simulink model "linearModel"  (R2019a)
settings: Solver=ode45  StartTime=0.0  StopTime=SimulationTime  MaxStep=maxstep  RelTol=rtol
undefined symbols (not defined in the file or in its folder): A, B, beta_operating, C, D, deviation, ePhi, operatingPoint
libraries: simulink x1
settings Model: Creator=000  LastModifiedBy=000

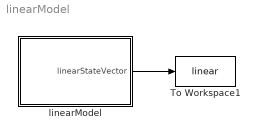
== system linearModel ==
  To Workspace1 : ToWorkspace  VariableName=linear  SaveFormat=Timeseries  SampleTime=-1
  linearModel : Subsystem
  wires:
  linearModel/1(linearStateVector) -> To Workspace1/1

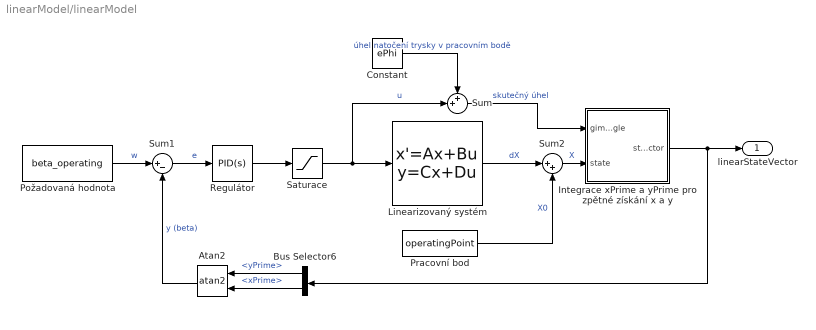
== system linearModel/linearModel ==
  Atan2 : Trigonometry  Operator=atan2
  Bus Selector6 : BusSelector  OutputSignals=yPrime,xPrime
  Constant : Constant  Value=ePhi
  Integrace xPrime a yPrime pro zpětné získání x a y : Subsystem
  Linearizovaný systém : StateSpace  A=A  B=B  C=C  D=D  InitialCondition=deviation
  Požadovaná hodnota : Constant  Value=beta_operating
  Pracovní bod : Constant  Value=operatingPoint
  Regulátor : simulink/Continuous/PID Controller  Controller=PID  Form=Parallel  TimeDomain=Continuous-time  SampleTime=-1  IntegratorMethod=Forward Euler  FilterMethod=Forward Euler  ControllerParametersSource=internal  P=-4.14526530426782  I=-0.338776014838026  D=1.82151949632533  UseFilter=on  N=1.42272875210404  TunerSelectOption=Frequency Response Based  InitialConditionSource=internal  InitialConditionForIntegrator=0  InitialConditionForFilter=0  DifferentiatorICPrevScaledInput=0  ExternalReset=none  TrackingMode=off  Kt=1  LimitOutput=on  UpperSaturationLimit=pi/4-ePhi  LowerSaturationLimit=-pi/4-ePhi  LinearizeAsGain=on  AntiWindupMode=back-calculation  Kb=1  POutMin=[]  POutMax=[]  IOutMin=[]  IOutMax=[]  DOutMin=[]  DOutMax=[]  NOutMin=[]  NOutMax=[]  SumOutMin=[]  SumOutMax=[]  SaturationOutMin=[]  SaturationOutMax=[]  PParamMin=[]  PParamMax=[]  IParamMin=[]  IParamMax=[]  DParamMin=[]  DParamMax=[]  NParamMin=[]  NParamMax=[]  KbParamMin=[]  KbParamMax=[]  KtParamMin=[]  KtParamMax=[]  KbOutMin=[]  KbOutMax=[]  KtOutMin=[]  KtOutMax=[]  IntegratorOutMin=[]  IntegratorOutMax=[]  FilterOutMin=[]  FilterOutMax=[]  SumI1OutMin=[]  SumI1OutMax=[]  SumI2OutMin=[]  SumI2OutMax=[]  SumI3OutMin=[]  SumI3OutMax=[]  SumI4OutMin=[]  SumI4OutMax=[]  SumDOutMin=[]  SumDOutMax=[]  DifferentiatorOutMin=[]  DifferentiatorOutMax=[]  FilterDiffOutCoefMin=[]  FilterDiffOutCoefMax=[]  ReciprocalOutMin=[]  ReciprocalOutMax=[]  SumDenOutMin=[]  SumDenOutMax=[]  SumNumOutMin=[]  SumNumOutMax=[]  DivideOutMin=[]  DivideOutMax=[]  IntegratorContinuousStateAttributes=''  IntegratorStateMustResolveToSignalObject=off  IntegratorRTWStateStorageClass=Auto  FilterContinuousStateAttributes=''  FilterStateMustResolveToSignalObject=off  FilterRTWStateStorageClass=Auto  ParallelPVariant=InternalParameters  IdealPVariant=Disabled  IVariant=InternalParameters  DVariant=InternalParameters  IntegratorVariant=Continuous  SatVariant=Enabled  AWVariant=BackCalculation  PCopyVariant=Disabled  TRVariant=Disabled  FdbkBlocksVariant=Forward  IdealPFdbkVariant=Disabled  SatFdbkVariant=Disabled  DerivativeFilterVariant=ContFilter  NVariant=InternalParameters  NCopyVariant=Disabled  FilterICVariant=InternalICsFilter  IntegratorICVariant=InternalICs  ExternalResetVariant=Disabled  TRSumVariant=Passthrough  SumFdbkVariant=Disabled  SumVariant=Sum_PID
  Saturace : Saturate  UpperLimit=pi/4-ePhi  LowerLimit=-pi/4-ePhi
  Sum : Sum  Inputs=++|
  Sum1 : Sum  Inputs=|+-
  Sum2 : Sum  Inputs=|++
  linearStateVector : Outport
  wires:
  Pracovní bod/1 -> Sum2/2  "X0"
  Saturace/1 -> Linearizovaný systém/1, Sum/2  "u"
  Bus Selector6/2 -> Atan2/2  "<xPrime>"
  Atan2/1 -> Sum1/2  "y (beta)"
  Sum1/1 -> Regulátor/1  "e"
  Bus Selector6/1 -> Atan2/1  "<yPrime>"
  Regulátor/1 -> Saturace/1
  Linearizovaný systém/1 -> Sum2/1  "dX"
  Integrace xPrime a yPrime pro zpětné získání x a y/1(stateVector) -> linearStateVector/1, Bus Selector6/1
  Sum2/1 -> Integrace xPrime a yPrime pro zpětné získání x a y/2(state)  "X"
  Požadovaná hodnota/1 -> Sum1/1  "w"
  Constant/1 -> Sum/1  "úhel natočení trysky v pracovním bodě"
  Sum/1 -> Integrace xPrime a yPrime pro zpětné získání x a y/1(gimbalAngle)  "skutečný úhel"

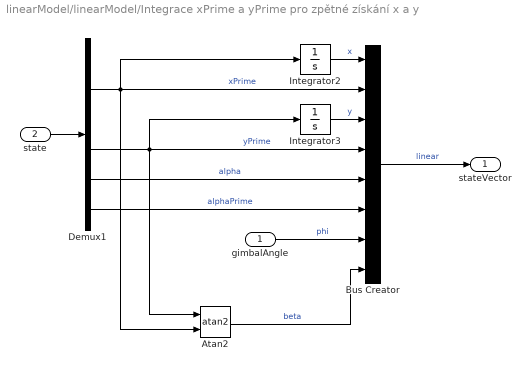
== system linearModel/linearModel/Integrace xPrime a yPrime pro zpětné získání x a y ==
  gimbalAngle : Inport
  state : Inport  Port=2
  Atan2 : Trigonometry  Operator=atan2
  Bus Creator : BusCreator  Inputs=8
  Demux1 : Demux  Outputs=6
  Integrator2 : Integrator
  Integrator3 : Integrator
  stateVector : Outport
  wires:
  Demux1/4 -> Bus Creator/4, Integrator3/1, Atan2/1  "yPrime"
  Demux1/2 -> Bus Creator/2, Integrator2/1, Atan2/2  "xPrime"
  Bus Creator/1 -> stateVector/1  "linear"
  Integrator2/1 -> Bus Creator/1  "x"
  Integrator3/1 -> Bus Creator/3  "y"
  Demux1/6 -> Bus Creator/6  "alphaPrime"
  Demux1/5 -> Bus Creator/5  "alpha"
  state/1 -> Demux1/1
  gimbalAngle/1 -> Bus Creator/7  "phi"
  Atan2/1 -> Bus Creator/8  "beta"
